simulink model "WaermeFlussSpindelTKonstant"  (Simulink 7.6)
settings: Solver=ode45  StartTime=0.0  StopTime="SimulTime "  RelTol=1e-6
undefined symbols (not defined in the file): A, f3, geometrie, KinematischeViskositaet, Pr, sb, Temperatur, Waermeleitfaehigkeit
settings Model: Creator=conid  LastModifiedBy=conid

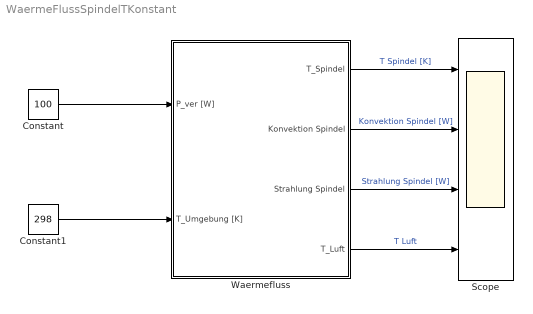
== system WaermeFlussSpindelTKonstant ==
  Constant : Constant  Value=100
  Constant1 : Constant  Value=298
  Scope : Scope  NumInputPorts=4
      settings: YMin=-5~-5~-5~-5  YMax=5~5~5~5  SaveName=Scp_HeatFlow
  Waermefluss : Subsystem  TreatAsAtomicUnit=on
  wires:
  Constant/1 -> Waermefluss/1(P_ver [W])
  Constant1/1 -> Waermefluss/2(T_Umgebung [K])
  Waermefluss/1(T_Spindel) -> Scope/1  "T Spindel [K]"
  Waermefluss/2(Konvektion Spindel) -> Scope/2  "Konvektion Spindel [W]"
  Waermefluss/3(Strahlung Spindel) -> Scope/3  "Strahlung Spindel [W]"
  Waermefluss/4(T_Luft) -> Scope/4  "T Luft"

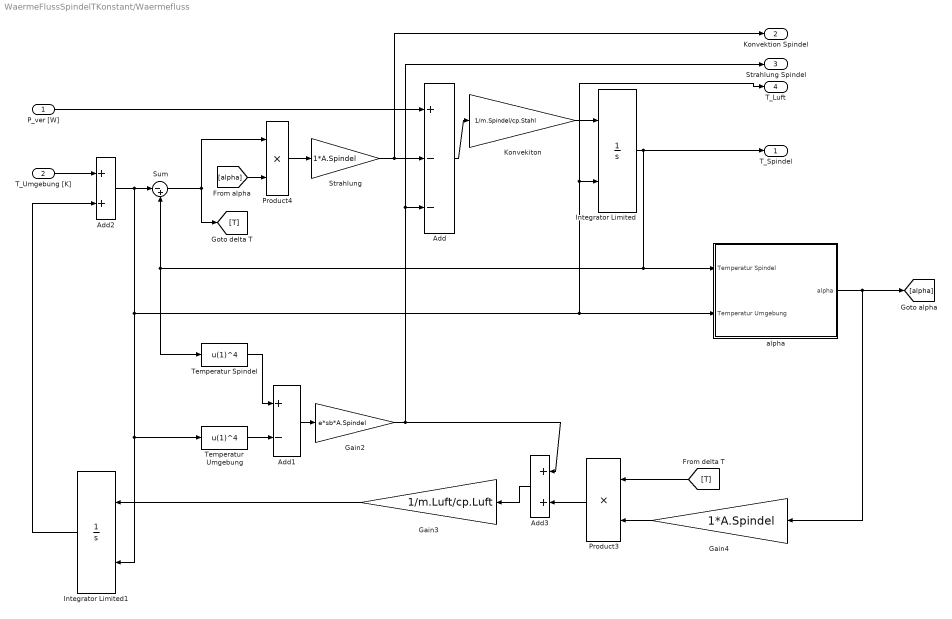
== system WaermeFlussSpindelTKonstant/Waermefluss ==
  P_ver [W] : Inport
  T_Umgebung [K] : Inport  Port=2
  Add : Sum  Inputs=+--
  Add1 : Sum  Inputs=+-
  Add2 : Sum
  Add3 : Sum
  Gain2 : Gain  Gain=e*sb*A.Spindel
  Gain3 : Gain  Gain=1/m.Luft/cp.Luft
  Gain4 : Gain  Gain=1*A.Spindel
  Integrator Limited : Integrator  InitialConditionSource=external  LimitOutput=on  ZeroCross=off
  Integrator Limited1 : Integrator  InitialConditionSource=external  LimitOutput=on  ZeroCross=off
  Konvekiton : Gain  Gain=1/m.Spindel/cp.Stahl
  Product3 : Product  RndMeth=Zero
  Product4 : Product  RndMeth=Zero
  Strahlung : Gain  Gain=1*A.Spindel
  Sum : Sum  Inputs=|-+
  Temperatur Spindel : Fcn  Expr=u(1)^4
  Temperatur Umgebung : Fcn  Expr=u(1)^4
  alpha : Subsystem
  T_Spindel : Outport
  Konvektion Spindel : Outport  Port=2
  Strahlung Spindel : Outport  Port=3
  T_Luft : Outport  Port=4
  wires:
  P_ver [W]/1 -> Add/1
  Sum/1 -> Product4/1, [T]
  Konvekiton/1 -> Integrator Limited/1
  Strahlung/1 -> Add/2, Konvektion Spindel/1
  Integrator Limited/1 -> Sum/2, Temperatur Spindel/1, T_Spindel/1, alpha/1(Temperatur Spindel)
  Add/1 -> Konvekiton/1
  Gain2/1 -> Strahlung Spindel/1, Add/3, Add3/1
  Temperatur Spindel/1 -> Add1/1
  Temperatur Umgebung/1 -> Add1/2
  Add1/1 -> Gain2/1
  Add2/1 -> Sum/1, Integrator Limited/2, T_Luft/1, alpha/2(Temperatur Umgebung), Temperatur Umgebung/1, Integrator Limited1/2
  T_Umgebung [K]/1 -> Add2/1
  Product4/1 -> Strahlung/1
  Gain3/1 -> Integrator Limited1/1
  [alpha] -> Product4/2
  Gain4/1 -> Product3/2
  [T] -> Product3/1
  alpha/1(alpha) -> [alpha], Gain4/1
  Product3/1 -> Add3/2
  Add3/1 -> Gain3/1
  Integrator Limited1/1 -> Add2/2

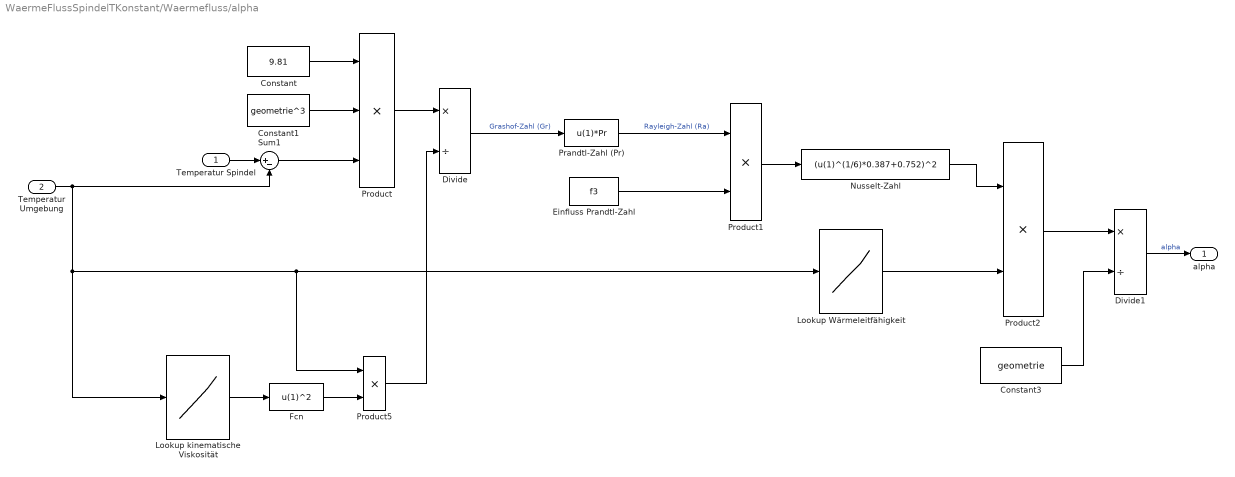
== system WaermeFlussSpindelTKonstant/Waermefluss/alpha ==
  Temperatur Spindel : Inport
  Temperatur Umgebung : Inport  Port=2
  Constant : Constant  Value=9.81
  Constant1 : Constant  Value=geometrie^3
  Constant3 : Constant  Value=geometrie
  Divide : Product  Inputs=*/
  Divide1 : Product  Inputs=*/
  Einfluss Prandtl-Zahl : Constant  Value=f3
  Fcn : Fcn  Expr=u(1)^2
  Lookup Wärmeleitfähigkeit : Lookup_n-D  NumberOfTableDimensions=1  BreakpointsForDimension1=Temperatur.Tabel  Table=Waermeleitfaehigkeit.Tabel  InterpMethod=Cubic spline  ExtrapMethod=None - Clip  InputSameDT=on
  Lookup kinematische Viskosität : Lookup_n-D  NumberOfTableDimensions=1  BreakpointsForDimension1=Temperatur.Tabel  Table=KinematischeViskositaet.Tabel  InterpMethod=Cubic spline  ExtrapMethod=None - Clip  InputSameDT=on
  Nusselt-Zahl : Fcn  Expr=(u(1)^(1/6)*0.387+0.752)^2
  Prandtl-Zahl (Pr) : Fcn  Expr=u(1)*Pr
  Product : Product  Inputs=3  RndMeth=Zero
  Product1 : Product  RndMeth=Zero
  Product2 : Product  RndMeth=Zero
  Product5 : Product  RndMeth=Zero
  Sum1 : Sum  Inputs=|+-
  alpha : Outport
  wires:
  Constant/1 -> Product/1
  Constant1/1 -> Product/2
  Sum1/1 -> Product/3
  Product/1 -> Divide/1
  Divide/1 -> Prandtl-Zahl (Pr)/1  "Grashof-Zahl (Gr)"
  Prandtl-Zahl (Pr)/1 -> Product1/1  "Rayleigh-Zahl (Ra)"
  Einfluss Prandtl-Zahl/1 -> Product1/2
  Lookup Wärmeleitfähigkeit/1 -> Product2/2
  Product2/1 -> Divide1/1
  Divide1/1 -> alpha/1  "alpha"
  Product5/1 -> Divide/2
  Lookup kinematische Viskosität/1 -> Fcn/1
  Fcn/1 -> Product5/2
  Product1/1 -> Nusselt-Zahl/1
  Nusselt-Zahl/1 -> Product2/1
  Constant3/1 -> Divide1/2
  Temperatur Spindel/1 -> Sum1/1
  Temperatur Umgebung/1 -> Lookup kinematische Viskosität/1, Product5/1, Lookup Wärmeleitfähigkeit/1, Sum1/2
